simulink model "rst"  (R2017b)
settings: Solver=VariableStepAuto  StartTime=0.0  StopTime=100  RelTol=1e-3
settings Model: Creator=AK47  LastModifiedBy=AK47
settings OptimizationCC: DefaultParameterBehavior=Inlined  UseDivisionForNetSlopeComputation=on  UseFloatMulNetSlope=on  InlineInvariantSignals=on  PassReuseOutputArgsAs=Individual arguments  ZeroExternalMemoryAtStartup=off  ZeroInternalMemoryAtStartup=off  NoFixptDivByZeroProtection=on  EfficientFloat2IntCast=on  LifeSpan=1
settings DebuggingCC: ParameterTunabilityLossMsg=error
settings HardwareCC: ProdBitPerPointer=32  ProdBitPerSizeT=32  ProdBitPerPtrDiffT=32  ProdLargestAtomicInteger=Long  ProdLargestAtomicFloat=Double  ProdWordSize=32  ProdLongLongMode=on  ProdHWDeviceType=NXP->Cortex-M4
settings SFSimCC: MATLABDynamicMemAlloc=off
settings RTWCC: SystemTargetFile=ert.tlc  TemplateMakefile=ert_default_tmf  GenerateReport=on  IncludeHyperlinkInReport=on  LaunchReport=on  GenerateTraceInfo=on  GenerateTraceReport=on  GenerateTraceReportSl=on  GenerateTraceReportSf=on  GenerateTraceReportEml=on  GenerateCodeMetricsReport=on
settings CodeAppCC: ForceParamTrailComments=on  IgnoreCustomStorageClasses=off  OperatorAnnotations=on  SimulinkDataObjDesc=on  SFDataObjDesc=on  CustomSymbolStrGlobalVar=rt$N$M  CustomSymbolStrType=$N$M  CustomSymbolStrFcn=$N$M$F  CustomSymbolStrMacro=$N$M  InsertBlockDesc=on
settings ERTTargetCC: TargetLangStandard=C99 (ISO)  GenerateSampleERTMain=on  IncludeMdlTerminateFcn=off  CombineSignalStateStructs=on  SupportComplex=off  InlinedParameterPlacement=NonHierarchical  ERTCustomFileTemplate=example_file_process.tlc  ERTFilePackagingFormat=CompactWithDataFile

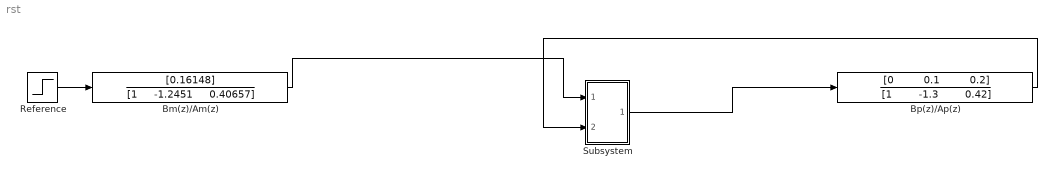
== system rst ==
  Bm(z)/Am(z) : DiscreteFilter  Numerator=[0.16148]  Denominator="[1     -1.2451     0.40657]"  SampleTime=1
  Bp(z)/Ap(z) : DiscreteFilter  Numerator="[0         0.1         0.2]"  Denominator="[1        -1.3        0.42]"  SampleTime=1
  Reference : Step  Time=5  SampleTime=1
  Subsystem : Subsystem
  wires:
  Reference/1 -> Bm(z)/Am(z)/1
  Bm(z)/Am(z)/1 -> Subsystem/1(In1)
  Bp(z)/Ap(z)/1 -> Subsystem/2(In2)
  Subsystem/1(Out1) -> Bp(z)/Ap(z)/1

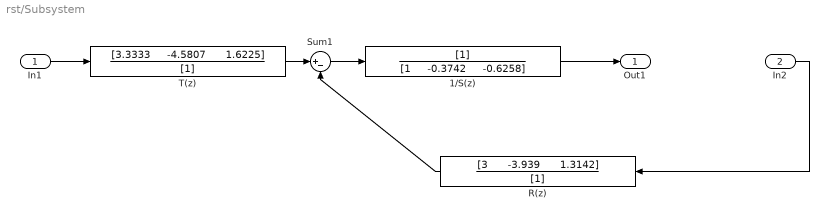
== system rst/Subsystem ==
  In1 : Inport
  In2 : Inport  Port=2
  1/S(z) : DiscreteFilter  Denominator="[1     -0.3742     -0.6258]"  SampleTime=1
  R(z) : DiscreteFilter  Numerator="[3      -3.939      1.3142]"  Denominator=[1]  SampleTime=1
  Sum1 : Sum  Inputs=|+-
  T(z) : DiscreteFilter  Numerator="[3.3333     -4.5807      1.6225]"  Denominator=[1]  SampleTime=1
  Out1 : Outport
  wires:
  In1/1 -> T(z)/1
  T(z)/1 -> Sum1/1
  Sum1/1 -> 1/S(z)/1
  1/S(z)/1 -> Out1/1
  In2/1 -> R(z)/1
  R(z)/1 -> Sum1/2
